simulink model "four_channel_bilateral_teleoperation_local_force"  (R2020b)
settings: Solver=VariableStepAuto  StartTime=0.0  StopTime=5  RelTol=1e-3
values from neighbouring files (symbols this model uses):
  A = 1    [Assignment_2.m]    (also in Assignment_2_discrete.m = [1 Ts)
  Be = 0    [Assignment_2.m]    (also in Assignment_2_discrete.m = 10)
  Bh = 70    [Assignment_2.m]    (also in Assignment_2_discrete.m)
  Bm = 0.8*100    (= 80)    [Assignment_2.m]    (also in Assignment_2_discrete.m = 144)
  Bs = 0.8*4*2    (= 6.4)    [Assignment_2.m]    (also in Assignment_2_discrete.m)
  Cmf = 0.6    [Assignment_2.m]    (also in Assignment_2_discrete.m)
  Csf = 0.6    [Assignment_2.m]    (also in Assignment_2_discrete.m)
  Dh = 100    [Assignment_2.m]    (also in Assignment_2_discrete.m)
  Dm = 0    [Assignment_2.m]    (also in Assignment_2_discrete.m)
  Ds = 0    [Assignment_2.m]    (also in Assignment_2_discrete.m)
  Fc = 1    [Assignment_2.m]    (also in Assignment_2_discrete.m)
  Fip = 1    [Assignment_2.m]    (also in Assignment_2_discrete.m)
  Je = 0    [Assignment_2.m]    (also in Assignment_2_discrete.m)
  Jh = 0.5    [Assignment_2.m]    (also in Assignment_2_discrete.m)
  Ke = 20    [Assignment_2.m]    (also in Assignment_2_discrete.m)
  Kh = 2000    [Assignment_2.m]    (also in Assignment_2_discrete.m)
  Km = 1*100    (= 100)    [Assignment_2.m]    (also in Assignment_2_discrete.m = 180)
  Ks = 4*2    (= 8)    [Assignment_2.m]    (also in Assignment_2_discrete.m)
  Mm = 0.5    [Assignment_2.m]    (also in Assignment_2_discrete.m)
  Ms = 2    [Assignment_2.m]    (also in Assignment_2_discrete.m)
  Ph = 200000    [Assignment_2.m]    (also in Assignment_2_discrete.m = 20000)
  tau = 10000    [Assignment_2.m]    (also in Assignment_2_discrete.m)
settings Model: Creator=anuj  LastModifiedBy=Edoardo

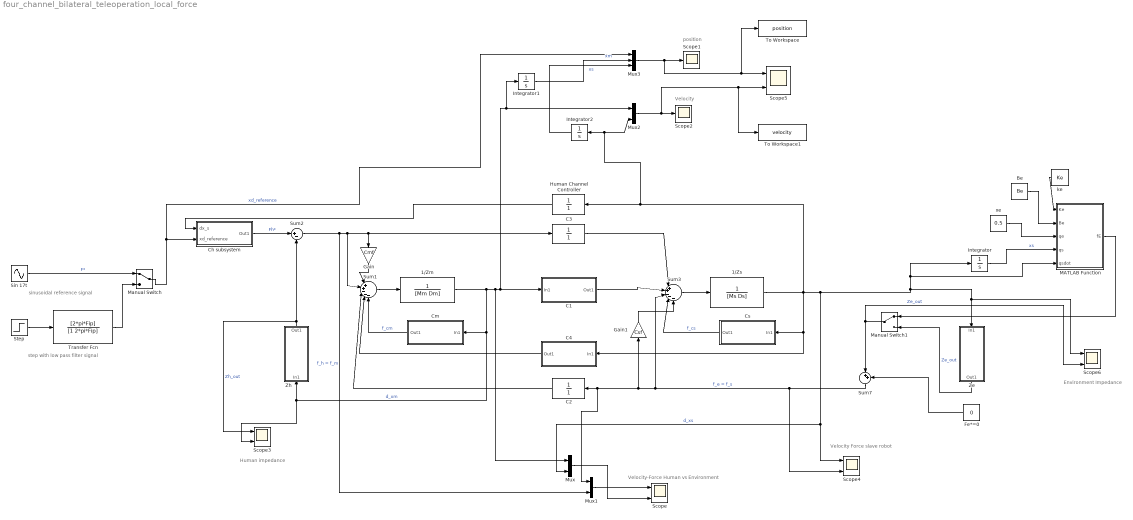
== system four_channel_bilateral_teleoperation_local_force ==
  note: Environment Impedance
  note: Human impedance
  note: Velocity-Force Human vs Environment
  note: Velocity Force slave robot
  note: sinusoidal reference signal
  note: step with low pass filter signal
  note: position
  note: Velocity
  1/Zm : TransferFcn  Denominator=[Mm Dm]
  1/Zs : TransferFcn  Denominator=[Ms Ds]
  Be : Constant  Value=Be
  C1 : Subsystem
  C2 : TransferFcn  Denominator=[1]
  C3 : TransferFcn  Denominator=[1]
  C4 : Subsystem
  Ch subsystem : Subsystem
  Cm : Subsystem
  Cs : Subsystem
  Fe*=0 : Constant  Value=0
  Gain : Gain  Gain=Cmf
  Gain1 : Gain  Gain=Csf
  Human Channel Controller : TransferFcn  Denominator=[1]
  Integrator : Integrator
  Integrator1 : Integrator
  Integrator2 : Integrator
  MATLAB Function : MATLAB Function  TreatAsAtomicUnit=on
  Manual Switch : ManualSwitch
  Manual Switch1 : ManualSwitch
  Mux : Mux  Inputs=2
  Mux1 : Mux  Inputs=2
  Mux2 : Mux  Inputs=2
  Mux3 : Mux  Inputs=3
  Scope{,3..6} (5 alike) : Scope  NumInputPorts=2
  Scope1 : Scope
  Scope2 : Scope
  Sin 17t : Sin  Amplitude=A  Frequency=2*pi*Fc  SampleTime=0
  Step : Step  After=A  SampleTime=0
  Sum1 : Sum  Inputs=|++---
  Sum2 : Sum  Inputs=|+-
  Sum3 : Sum  Inputs=|++---
  Sum7 : Sum  Inputs=|++
  To Workspace : ToWorkspace  VariableName=position  SaveFormat=Timeseries  SampleTime=-1
  To Workspace1 : ToWorkspace  VariableName=velocity  SaveFormat=Timeseries  SampleTime=-1
  Transfer Fcn : TransferFcn  Numerator=[2*pi*Fip]  Denominator=[1 2*pi*Fip]
  Ze : Subsystem
  Zh : Subsystem
  ke : Constant  Value=Ke
  xe : Constant  Value=0.5
  wires:
  Mux/1 -> Scope/2
  Mux1/1 -> Scope/1
  Sum2/1 -> C3/1, Gain/1, Sum1/2, Mux1/2  "f_h = f_m"
  1/Zm/1 -> Mux2/1, Integrator1/1, C1/1(In1), Mux/1, Zh/1(In1), Scope3/2, Cm/1(In1)  "d_xm"
  Sum1/1 -> 1/Zm/1
  C2/1 -> Sum1/3
  C3/1 -> Sum3/1
  Sum3/1 -> 1/Zs/1
  Fe*=0/1 -> Sum7/2
  Sum7/1 -> Sum3/3, Gain1/1, Mux1/1, C2/1, Scope4/2  "f_e = f_s"
  C4/1(Out1) -> Sum1/4
  Ch subsystem/1(Out1) -> Sum2/1  "Fh*"
  Be/1 -> MATLAB Function/2(Be)
  xe/1 -> MATLAB Function/3(qe)
  ke/1 -> MATLAB Function/1(Ke)
  Integrator/1 -> MATLAB Function/4(qs)  "xs"
  Transfer Fcn/1 -> Manual Switch/2
  Step/1 -> Transfer Fcn/1
  Human Channel Controller/1 -> Ch subsystem/1(dx_s)
  Manual Switch/1 -> Mux3/1, Ch subsystem/2(xd_reference)  "xd_reference"
  Sin 17t/1 -> Manual Switch/1  "F*"
  C1/1(Out1) -> Sum3/2
  MATLAB Function/1(fE) -> Manual Switch1/1
  Manual Switch1/1 -> Sum7/1, Scope6/2  "Ze_out"
  Zh/1(Out1) -> Sum2/2, Scope3/1  "Zh_out"
  Cm/1(Out1) -> Sum1/5  "f_cm"
  Cs/1(Out1) -> Sum3/4  "f_cs"
  Ze/1(Out1) -> Manual Switch1/2  "Ze_out"
  Gain/1 -> Sum1/1
  Gain1/1 -> Sum3/5
  Mux3/1 -> Scope1/1, To Workspace/1, Scope5/1
  Integrator1/1 -> Mux3/2  "xm"
  Integrator2/1 -> Mux3/3  "xs"
  Mux2/1 -> Scope2/1, To Workspace1/1, Scope5/2
  1/Zs/1 -> Integrator2/1, Mux2/2, Human Channel Controller/1, Scope4/1, Mux/2, MATLAB Function/5(qsdot), Integrator/1, Scope6/1, Ze/1(In1), C4/1(In1), Cs/1(In1)  "d_xs"

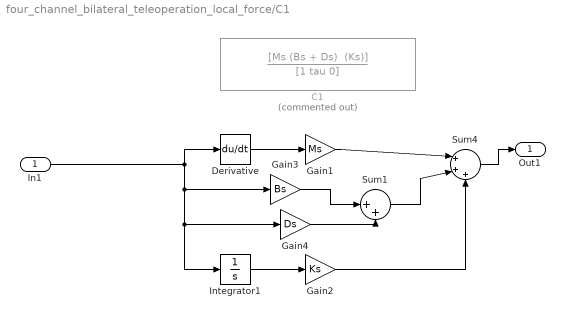
== system four_channel_bilateral_teleoperation_local_force/C1 ==
  In1 : Inport
  C1 : TransferFcn  Commented=on  Numerator="[Ms (Bs + Ds)  (Ks)]"  Denominator=[1 tau 0]
  Derivative : Derivative
  Gain1 : Gain  Gain=Ms
  Gain2 : Gain  Gain=Ks
  Gain3 : Gain  Gain=Bs
  Gain4 : Gain  Gain=Ds
  Integrator1 : Integrator
  Sum1 : Sum  Inputs=|++
  Sum4 : Sum  Inputs=|+++
  Out1 : Outport
  wires:
  Sum4/1 -> Out1/1
  Gain1/1 -> Sum4/1
  Integrator1/1 -> Gain2/1
  In1/1 -> Derivative/1, Gain3/1, Gain4/1, Integrator1/1
  Gain2/1 -> Sum4/3
  Sum1/1 -> Sum4/2
  Gain3/1 -> Sum1/1
  Derivative/1 -> Gain1/1
  Gain4/1 -> Sum1/2

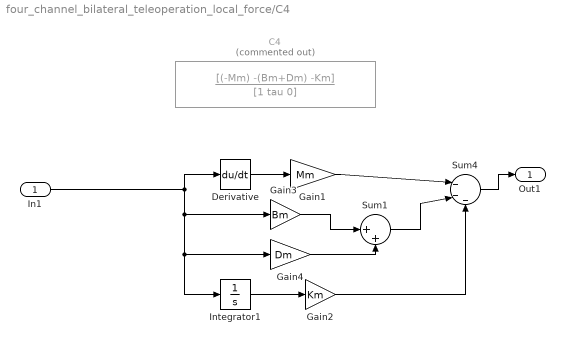
== system four_channel_bilateral_teleoperation_local_force/C4 ==
  In1 : Inport
  C4 : TransferFcn  Commented=on  Numerator=[(-Mm) -(Bm+Dm) -Km]  Denominator=[1 tau 0]
  Derivative : Derivative
  Gain1 : Gain  Gain=Mm
  Gain2 : Gain  Gain=Km
  Gain3 : Gain  Gain=Bm
  Gain4 : Gain  Gain=Dm
  Integrator1 : Integrator
  Sum1 : Sum  Inputs=|++
  Sum4 : Sum  Inputs=|---
  Out1 : Outport
  wires:
  Sum4/1 -> Out1/1
  Gain1/1 -> Sum4/1
  Integrator1/1 -> Gain2/1
  In1/1 -> Derivative/1, Gain3/1, Integrator1/1, Gain4/1
  Gain2/1 -> Sum4/3
  Sum1/1 -> Sum4/2
  Gain4/1 -> Sum1/2
  Gain3/1 -> Sum1/1
  Derivative/1 -> Gain1/1

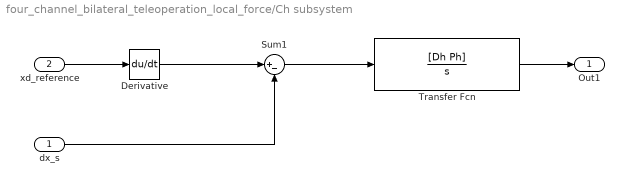
== system four_channel_bilateral_teleoperation_local_force/Ch subsystem ==
  dx_s : Inport
  xd_reference : Inport  Port=2
  Derivative : Derivative
  Sum1 : Sum  Inputs=|+-
  Transfer Fcn : TransferFcn  Numerator=[Dh Ph]  Denominator=[1 0]
  Out1 : Outport
  wires:
  dx_s/1 -> Sum1/2
  Sum1/1 -> Transfer Fcn/1
  xd_reference/1 -> Derivative/1
  Derivative/1 -> Sum1/1
  Transfer Fcn/1 -> Out1/1

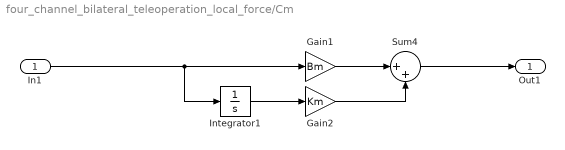
== system four_channel_bilateral_teleoperation_local_force/Cm ==
  In1 : Inport
  Gain1 : Gain  Gain=Bm
  Gain2 : Gain  Gain=Km
  Integrator1 : Integrator
  Sum4 : Sum  Inputs=|++
  Out1 : Outport
  wires:
  Sum4/1 -> Out1/1
  Gain1/1 -> Sum4/1
  Integrator1/1 -> Gain2/1
  In1/1 -> Gain1/1, Integrator1/1
  Gain2/1 -> Sum4/2

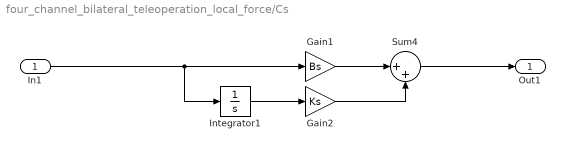
== system four_channel_bilateral_teleoperation_local_force/Cs ==
  In1 : Inport
  Gain1 : Gain  Gain=Bs
  Gain2 : Gain  Gain=Ks
  Integrator1 : Integrator
  Sum4 : Sum  Inputs=|++
  Out1 : Outport
  wires:
  Sum4/1 -> Out1/1
  Gain1/1 -> Sum4/1
  Integrator1/1 -> Gain2/1
  In1/1 -> Gain1/1, Integrator1/1
  Gain2/1 -> Sum4/2

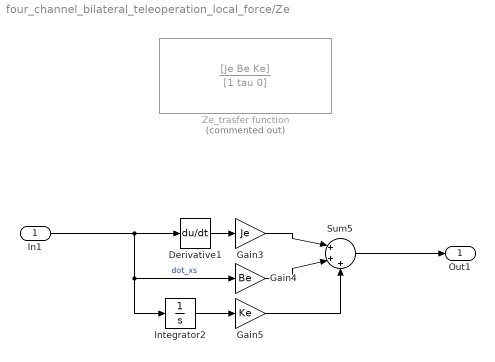
== system four_channel_bilateral_teleoperation_local_force/Ze ==
  In1 : Inport
  Derivative1 : Derivative
  Gain3 : Gain  Gain=Je
  Gain4 : Gain  Gain=Be
  Gain5 : Gain  Gain=Ke
  Integrator2 : Integrator
  Sum5 : Sum  Inputs=|+++
  Ze_trasfer function : TransferFcn  Commented=on  Numerator=[Je Be Ke]  Denominator=[1 tau 0]
  Out1 : Outport
  wires:
  Gain4/1 -> Sum5/2
  Gain3/1 -> Sum5/1
  Gain5/1 -> Sum5/3
  Sum5/1 -> Out1/1
  Integrator2/1 -> Gain5/1
  In1/1 -> Integrator2/1, Gain4/1, Derivative1/1  "dot_xs"
  Derivative1/1 -> Gain3/1

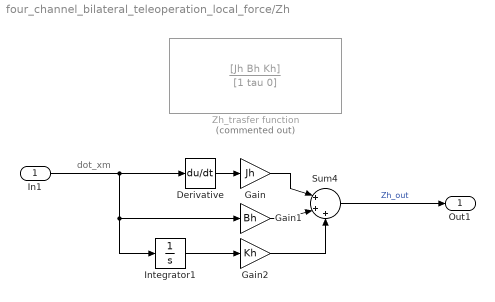
== system four_channel_bilateral_teleoperation_local_force/Zh ==
  note: dot_xm
  In1 : Inport
  Derivative : Derivative
  Gain : Gain  Gain=Jh
  Gain1 : Gain  Gain=Bh
  Gain2 : Gain  Gain=Kh
  Integrator1 : Integrator
  Sum4 : Sum  Inputs=|+++
  Zh_trasfer function : TransferFcn  Commented=on  Numerator=[Jh Bh Kh]  Denominator=[1 tau 0]
  Out1 : Outport
  wires:
  Derivative/1 -> Gain/1
  Integrator1/1 -> Gain2/1
  Gain2/1 -> Sum4/3
  Gain1/1 -> Sum4/2
  Gain/1 -> Sum4/1
  Sum4/1 -> Out1/1  "Zh_out"
  In1/1 -> Gain1/1, Integrator1/1, Derivative/1

== matlab function four_channel_bilateral_teleoperation_local_force/MATLAB Function ==
  data: Ke input; fE output; Be input; qe input; qs input; qsdot input
function fE = environment(Ke, Be, qe, qs, qsdot)
    if qs > qe
        fE = Ke * (qs - qe) + Be * qsdot;
    else
        fE = 0;
    end
end
